simulink library "Lib_rotation_matrix"  (R2024b)
settings: Solver=VariableStepAuto  StartTime=0.0  StopTime=10.0  RelTol=1e-3
settings Model: Creator=stefa  LastModifiedBy=stefa

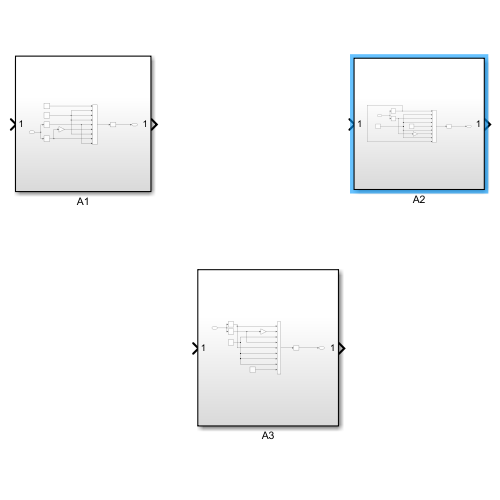
[thumbnail: Simulink's stored preview of the top-level diagram]
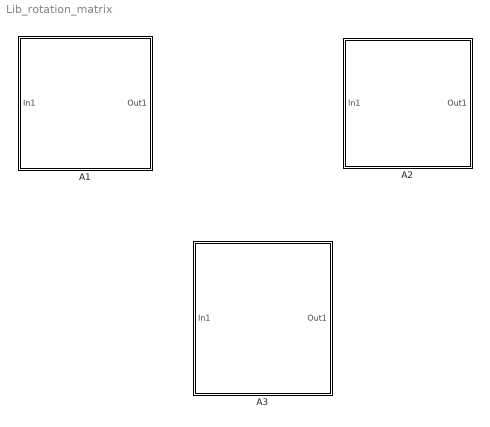
== system Lib_rotation_matrix ==
  A1 : Subsystem
  A2 : Subsystem
  A3 : Subsystem

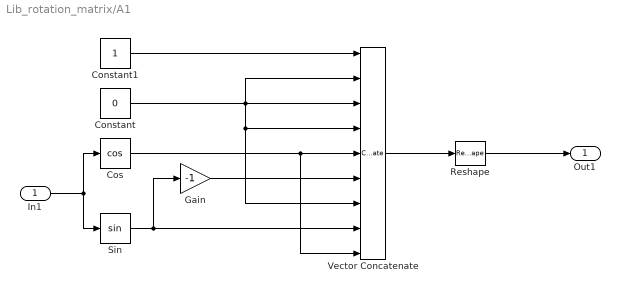
== system Lib_rotation_matrix/A1 ==
  In1 : Inport
  Constant : Constant  Value=0
  Constant1 : Constant
  Cos : Trigonometry  Operator=cos
  Gain : Gain  Gain=-1
  Reshape : Reshape  OutputDimensionality=Customize  OutputDimensions=[3,3]
  Sin : Trigonometry
  Vector Concatenate : Concatenate  NumInputs=9
  Out1 : Outport
  wires:
  In1/1 -> Sin/1, Cos/1
  Constant1/1 -> Vector Concatenate/1
  Constant/1 -> Vector Concatenate/7, Vector Concatenate/4, Vector Concatenate/3, Vector Concatenate/2
  Cos/1 -> Vector Concatenate/9, Vector Concatenate/5
  Vector Concatenate/1 -> Reshape/1
  Sin/1 -> Vector Concatenate/8, Gain/1
  Reshape/1 -> Out1/1
  Gain/1 -> Vector Concatenate/6

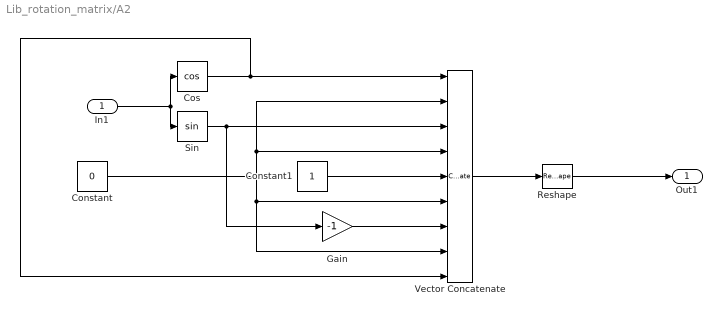
== system Lib_rotation_matrix/A2 ==
  In1 : Inport
  Constant : Constant  Value=0
  Constant1 : Constant
  Cos : Trigonometry  Operator=cos
  Gain : Gain  Gain=-1
  Reshape : Reshape  OutputDimensionality=Customize  OutputDimensions=[3,3]
  Sin : Trigonometry
  Vector Concatenate : Concatenate  NumInputs=9
  Out1 : Outport
  wires:
  Vector Concatenate/1 -> Reshape/1
  Constant/1 -> Vector Concatenate/6, Vector Concatenate/8, Vector Concatenate/4, Vector Concatenate/2
  Cos/1 -> Vector Concatenate/1, Vector Concatenate/9
  Reshape/1 -> Out1/1
  In1/1 -> Sin/1, Cos/1
  Sin/1 -> Vector Concatenate/3, Gain/1
  Constant1/1 -> Vector Concatenate/5
  Gain/1 -> Vector Concatenate/7

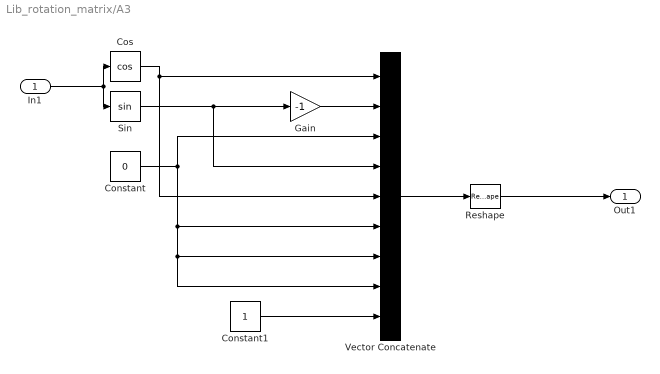
== system Lib_rotation_matrix/A3 ==
  In1 : Inport
  Constant : Constant  Value=0
  Constant1 : Constant
  Cos : Trigonometry  Operator=cos
  Gain : Gain  Gain=-1
  Reshape : Reshape  OutputDimensionality=Customize  OutputDimensions=[3,3]
  Sin : Trigonometry
  Vector Concatenate : Concatenate  NumInputs=9
  Out1 : Outport
  wires:
  In1/1 -> Sin/1, Cos/1
  Reshape/1 -> Out1/1
  Cos/1 -> Vector Concatenate/5, Vector Concatenate/1
  Constant1/1 -> Vector Concatenate/9
  Sin/1 -> Vector Concatenate/4, Gain/1
  Vector Concatenate/1 -> Reshape/1
  Constant/1 -> Vector Concatenate/8, Vector Concatenate/7, Vector Concatenate/6, Vector Concatenate/3
  Gain/1 -> Vector Concatenate/2
